simulink model "two"  (R2017a)
settings: Solver=VariableStepAuto  StartTime=0.0  StopTime=30  RelTol=1e-3
undefined symbols (not defined in the file): Cwy1, Cwy2, Jyy, k1_k, k2_k, K_thruster, kc, lambda55, T_thruster
settings Model: Creator=Eugene  LastModifiedBy=Eugene

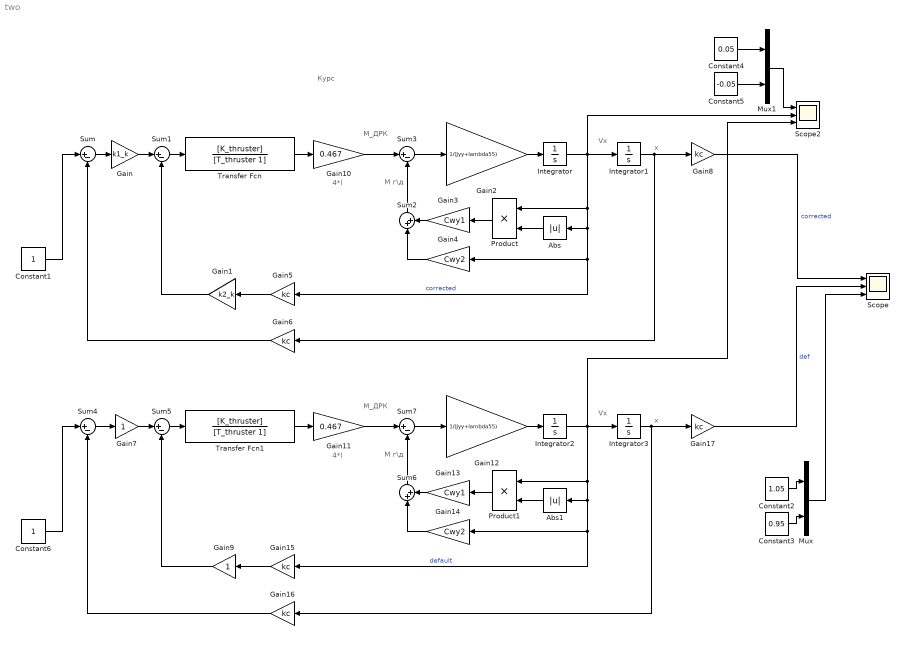
== system two ==
  note: M г\д
  note: M_ДРК
  note: Курс
  note: x
  note: Vx
  note: 4*l
  note: M г\д
  note: M_ДРК
  note: x
  note: Vx
  note: 4*l
  Abs : Abs
  Abs1 : Abs
  Constant1 : Constant
  Constant2 : Constant  Value=1.05
  Constant3 : Constant  Value=0.95
  Constant4 : Constant  Value=0.05
  Constant5 : Constant  Value=-0.05
  Constant6 : Constant
  Gain : Gain  Gain=k1_k
  Gain1 : Gain  Gain=k2_k
  Gain10 : Gain  Gain=0.467
  Gain11 : Gain  Gain=0.467
  Gain12 : Gain  Gain=1/(Jyy+lambda55)
  Gain13 : Gain  Gain=Cwy1
  Gain14 : Gain  Gain=Cwy2
  Gain{5..6,8,15..17} (6 alike) : Gain  Gain=kc
  Gain2 : Gain  Gain=1/(Jyy+lambda55)
  Gain3 : Gain  Gain=Cwy1
  Gain4 : Gain  Gain=Cwy2
  Gain7 : Gain
  Gain9 : Gain
  Integrator{,1..3} (4 alike) : Integrator
  Mux : Mux  Inputs=2
  Mux1 : Mux  Inputs=2
  Product : Product
  Product1 : Product
  Scope : Scope  NumInputPorts=3
  Scope2 : Scope  NumInputPorts=3
  Sum{,1,3..5,7} (6 alike) : Sum  Inputs=|+-
  Sum2 : Sum  Inputs=|++
  Sum6 : Sum  Inputs=|++
  Transfer Fcn : TransferFcn  Numerator=[K_thruster]  Denominator=[T_thruster 1]
  Transfer Fcn1 : TransferFcn  Numerator=[K_thruster]  Denominator=[T_thruster 1]
  wires:
  Constant1/1 -> Sum/1
  Sum/1 -> Gain/1
  Gain/1 -> Sum1/1
  Sum1/1 -> Transfer Fcn/1
  Gain2/1 -> Integrator/1
  Abs/1 -> Product/2
  Product/1 -> Gain3/1
  Sum3/1 -> Gain2/1
  Transfer Fcn/1 -> Gain10/1
  Gain1/1 -> Sum1/2
  Integrator/1 -> Gain5/1, Gain4/1, Abs/1, Product/1, Scope2/2, Integrator1/1  "corrected"
  Integrator1/1 -> Gain8/1, Gain6/1
  Gain10/1 -> Sum3/1
  Constant2/1 -> Mux/1
  Constant3/1 -> Mux/2
  Mux/1 -> Scope/3
  Mux1/1 -> Scope2/1
  Constant5/1 -> Mux1/2
  Constant4/1 -> Mux1/1
  Gain3/1 -> Sum2/2
  Sum2/1 -> Sum3/2
  Gain4/1 -> Sum2/1
  Gain5/1 -> Gain1/1
  Gain6/1 -> Sum/2
  Gain8/1 -> Scope/1  "corrected"
  Gain17/1 -> Scope/2  "def"
  Gain16/1 -> Sum4/2
  Gain15/1 -> Gain9/1
  Gain14/1 -> Sum6/1
  Sum6/1 -> Sum7/2
  Gain13/1 -> Sum6/2
  Gain11/1 -> Sum7/1
  Integrator3/1 -> Gain17/1, Gain16/1
  Integrator2/1 -> Scope2/3, Integrator3/1, Product1/1, Abs1/1, Gain14/1, Gain15/1  "default"
  Gain9/1 -> Sum5/2
  Transfer Fcn1/1 -> Gain11/1
  Sum7/1 -> Gain12/1
  Product1/1 -> Gain13/1
  Abs1/1 -> Product1/2
  Gain12/1 -> Integrator2/1
  Sum5/1 -> Transfer Fcn1/1
  Gain7/1 -> Sum5/1
  Sum4/1 -> Gain7/1
  Constant6/1 -> Sum4/1
